simulink model "state_machine"  (R2025b)
settings: Solver=VariableStepAuto  StartTime=0.0  StopTime=100.0  RelTol=1e-3
settings Model: Creator=hyper  LastModifiedBy=hyper

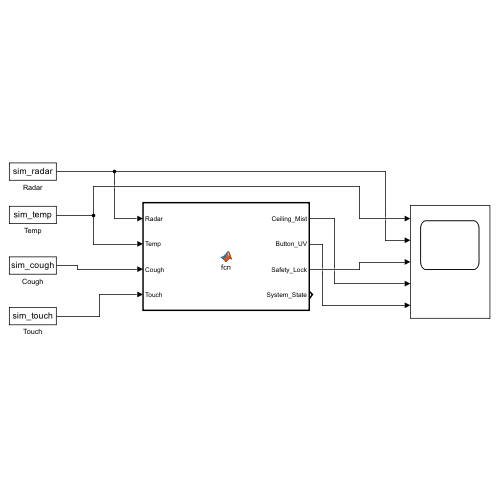
[thumbnail: Simulink's stored preview of the top-level diagram]
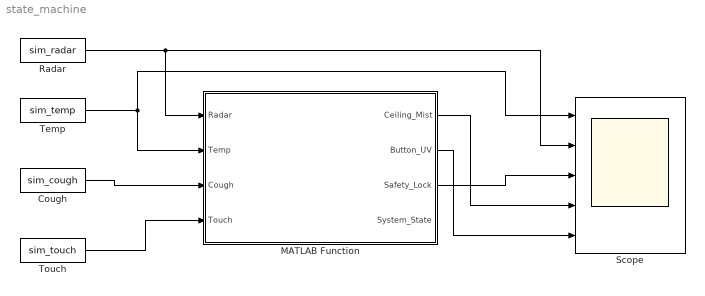
== system state_machine ==
  Cough : FromWorkspace  VariableName=sim_cough
  MATLAB Function : MATLAB Function  TreatAsAtomicUnit=on
  Radar : FromWorkspace  VariableName=sim_radar
  Scope : Scope  NumInputPorts=5
  Temp : FromWorkspace  VariableName=sim_temp
  Touch : FromWorkspace  VariableName=sim_touch
  wires:
  Radar/1 -> Scope/2, MATLAB Function/1(Radar)
  Temp/1 -> MATLAB Function/2(Temp), Scope/1
  Cough/1 -> MATLAB Function/3(Cough)
  Touch/1 -> MATLAB Function/4(Touch)
  MATLAB Function/3(Safety_Lock) -> Scope/3
  MATLAB Function/1(Ceiling_Mist) -> Scope/4
  MATLAB Function/2(Button_UV) -> Scope/5

== matlab function state_machine/MATLAB Function ==
  data: Radar input; Ceiling_Mist output; Temp input; Cough input; Touch input; Button_UV output; Safety_Lock output; System_State output
function [Ceiling_Mist, Button_UV, Safety_Lock, System_State] = fcn(Radar, Temp, Cough, Touch)
    % PATENT CONTROLLER LOGIC: "The Brain"
    % Implements State Machine + Safety Interlock + Targeted Cleaning
    
    % --- INTERNAL MEMORY ---
    persistent state max_temp cough_detected touched_buttons clean_timer_mist clean_timer_btn
    
    if isempty(state)
        state = 0;              % 0=IDLE, 1=MONITORING, 2=SANITIZING
        max_temp = 0;
        cough_detected = 0;
        touched_buttons = [0 0 0 0]; % Status of Buttons 1-4
        clean_timer_mist = 0;
        clean_timer_btn = 0;
    end
    
    % --- CONSTANTS ---
    FEVER_LIMIT = 37.8;
    MIST_TIME = 1000;    % 10 seconds (at 10ms steps)
    BTN_TIME = 500;      % 5 seconds
    
    % --- 1. SENSOR FUSION LAYER ---
    % Track highest threat level while passenger is inside
    if Radar > 0
        if Temp > max_temp
            max_temp = Temp;
        end
        if Cough > 0
            cough_detected = 1;
        end
        if Touch > 0
            % Mark specific button as "Touched"
            touched_buttons(Touch) = 1; 
        end
    end
    
    % --- 2. STATE MACHINE LAYER ---
    switch state
        case 0 % IDLE
            if Radar > 0
                state = 1; % Passenger Entered
            end
            
        case 1 % MONITORING (Passenger Inside)
            % SAFETY INTERLOCK: ABSOLUTE PRIORITY
            % While Radar=1, ALL Actuators must be clamped to 0
            if Radar == 0
                % Passenger Exit Detected -> DECISION GATE
                
                % LOGIC: Only clean if Fever OR Cough detected
                is_biohazard = (max_temp > FEVER_LIMIT) || (cough_detected > 0);
                
                if is_biohazard
                    state = 2; % Start Cleaning
                    clean_timer_mist = MIST_TIME;
                    clean_timer_btn = BTN_TIME;
                else
                    % Healthy Passenger -> Reset & Go to IDLE
                    state = 0;
                    max_temp = 0;
                    cough_detected = 0;
                    touched_buttons = [0 0 0 0];
                end
            end
            
        case 2 % SANITIZING (The "Cleaning Cycle")
            % Countdown Logic
            if clean_timer_mist > 0
                clean_timer_mist = clean_timer_mist - 1;
            end
            if clean_timer_btn > 0
                clean_timer_btn = clean_timer_btn - 1;
            end
            
            % Exit Condition
            if clean_timer_mist <= 0 && clean_timer_btn <= 0
                state = 0; % Done
                max_temp = 0;
                cough_detected = 0;
                touched_buttons = [0 0 0 0];
            end
            
            % EMERGENCY INTERRUPT
            % If someone re-enters during cleaning, STOP IMMEDIATELY
            if Radar > 0
                state = 1;
                clean_timer_mist = 0;
                clean_timer_btn = 0;
            end
    end
    
    % --- 3. ACTUATOR OUTPUT LAYER ---
    
    % Safety Lock Status (For Diagnostics)
    Safety_Lock = (Radar > 0);
    
    % Ceiling Mist Output
    if state == 2 && clean_timer_mist > 0
        Ceiling_Mist = 1;
    else
        Ceiling_Mist = 0;
    end
    
    % Button UV Output
    % Only activate if state is cleaning AND timer is running
    if state == 2 && clean_timer_btn > 0
        Button_UV = 1; 
    else
        Button_UV = 0;
    end
    
    % Debug State Output
    System_State = state;
end
